simulink library "SelectiveChannelMuteBtc"  (R2022b)
settings: Solver=VariableStepAuto  StartTime=0.0  StopTime=10.0  RelTol=1e-3
libraries: TuneVar x3, $bdroot x2, RTC x2, FeaturePath x1, HandyTextFile x1, RgainyBtc x1
settings Model: Creator=kl13806  LastModifiedBy=kl13806
settings SolverCC: AlgebraicLoopSolver=TrustRegion
settings DebuggingCC: UnconnectedInputMsg=warning  UnconnectedOutputMsg=warning  UnconnectedLineMsg=warning  SFMachineParentedDataDiag=warning
settings ModelReferenceCC: EnableRefExpFcnMdlSchedulingChecks=on
settings RTWCC: DLArmComputeVersion=19.05

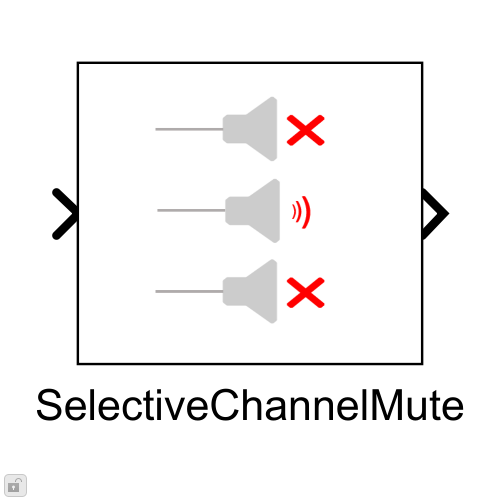
[thumbnail: Simulink's stored preview of the top-level diagram]
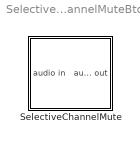
== system SelectiveChannelMuteBtc ==
  SelectiveChannelMute : Subsystem  mask(Bose Selective Channel Mute){Config=[], FeatureName=SCMute}
      mask prompts: Config "SelectiveChannelMuteConfig"; FeatureName "Feature path name:"
      mask help: This block offers the ability to mute individual channels selctively, by way of RGAINY and a "mute map". Set the initial mute state to a logical 1 (all channels muted) or 0 (no channels muted). There is runtime support via an RTC to selectively mute channels.
      mask init:
      | blkh=gcbh;
      | Config=BTConfig.Assert(blkh,Config);
      | Config.Validate();
      | BTConfig.InitSetFeatureIfPresent(blkh,'FeatureName');
      | 
      | 
      | MaskNumChannels = Config.NumChannelsIn;
      | 
      | % Set boundary conditions
      | rampRateBounds = [5,50000];
      | rampTimeBounds = [1,3000];
      mask Help:
      | This block offers the ability to mute individual channels seelctively, by way or RGAINY and a "mute map". Set the initial mute state to a logical 1 (all channels muted) or 0 (no channels muted). There is runtime support via an RTC to selectively mute channels.
      | 
      | RTC CONTROL:
      | Run time control is available to dynamically mute the audio of individual channels. The mute status can be provided to each channel through an array named "mute map". This array will be size 1 by numberOfInputChannels, and the elements of the array will be 1's (mute) or 0's (unmute), along with a ramp time and rate (rate gets precedence).
      | RTC_SIM_OBJ.AddREQ( 'SelectiveChannelMuteSet', 0.6, [0005,  <muteMap>, <ramp_db_per_second>, <ramp_time>]);
      | E.g., RTC_SIM_OBJ.AddREQ( 'MuteSet', 0.7, [0002, [1 0 0 1 0], 0, 50]);   % This message will mute channels 1 and 4 while keeping 2, 3, and 5 unmuted, all with a ramp time of 50 msec.
      mask Callback Config: BTConfig.CallbackHideIfPresent(gcbh,{'FeatureName'});
      mask TypeOptions FeatureName: FeaturePath/FeatureName
      mask Display: image('SCMuteIcon.png');

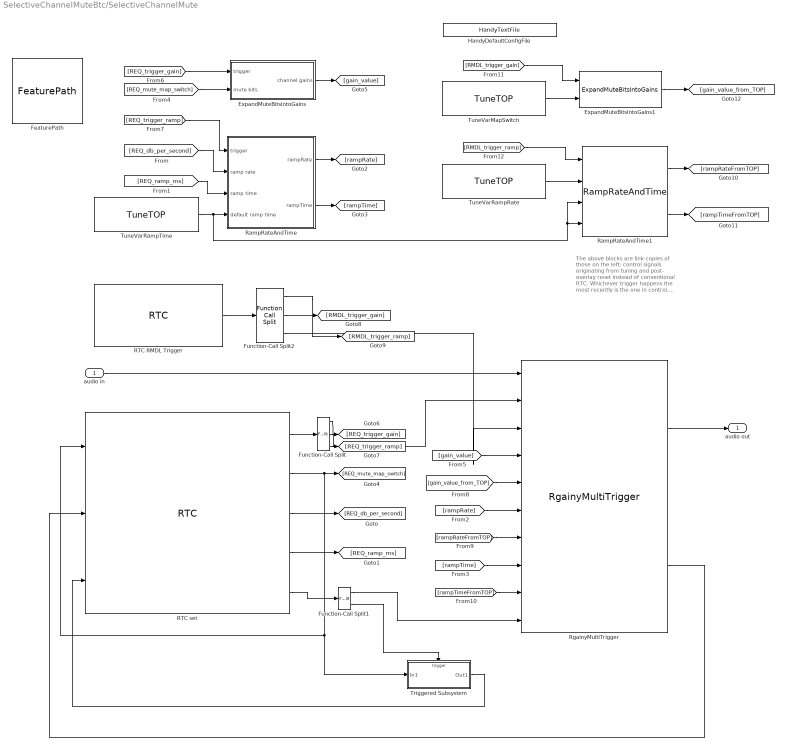
== system SelectiveChannelMuteBtc/SelectiveChannelMute ==
  note: The above blocks are link-copies
      | of those on the left: control signals
      | originating from tuning and post-
      | overlay reset instead of conventional
      | RTC. Whichever trigger happens the
      | most recently is the one in control.
      | (Note this design likely violates
      | standard RTC control assumptions)
  audio in : Inport
  ExpandMuteBitsIntoGains : Subsystem
  ExpandMuteBitsIntoGains1 : $bdroot/SelectiveChannelMute/ExpandMuteBitsIntoGains  SystemSampleTime=-1  VariantActivationTime=update diagram  Latency=0  AutoFrameSizeCalculation=off
  FeaturePath : FeaturePath/FeaturePath  FeatureName=SCMute  IsGroup=off  GroupNumber=-1  IsModule=off  TriggerInit=[20 -346 135 -239]
      settings: SourceProductName=Bose Talaria
  Function-Call Split : FunctionCallSplit  IconShape=distinctive  NumOutputPorts=3
  Function-Call Split1 : FunctionCallSplit  IconShape=distinctive  NumOutputPorts=2  OutputPortLayout=default
  Function-Call Split2 : FunctionCallSplit  IconShape=distinctive  NumOutputPorts=3
  HandyDefaultConfigFile : HandyTextFile/HandyTextFile  TemplateSource=Config  FileSuffix=Init  OpenDialogOnLoad=off  UseThisBlockName=off  AddGrandParentNamePrefix=off  TheDefaultText=|  ShowInLibBrowser=on
      | % $(FILENAME) Setup model parameters for each "Init" callback (e.g. update diagram)
      | sample_rate_in_hertz = 44100;
      | frame_size = 32;
      | sysin_channel_count = 2;
      settings: SourceProductName=Bose Talaria
  RTC RMDL Trigger : RTC/RTC  REQ_Priority=RTC_Mask.NormalPriority  RequestAtInit=off  EnableRequest=on  REQElemType1=uint32  REQElemWidth1=1  REQElemInitial1=[]  REQElemType2=uint32  REQElemWidth2=1  REQElemInitial2=[]  REQElemType3=uint32  REQElemWidth3=1  REQElemInitial3=[]  REQElemType4=uint32  REQElemWidth4=1  REQElemInitial4=[]  REQElemType5=uint32  REQElemWidth5=1  REQElemInitial5=[]  REQElemType6=uint32  REQElemWidth6=1  REQElemInitial6=[]  REQElemType7=uint32  REQElemWidth7=1  REQElemInitial7=[]  REQElemType8=uint32  REQElemWidth8=1  REQElemInitial8=[]  REQElemType9=uint32  REQElemWidth9=1  REQElemInitial9=[]  REQElemType10=uint32  REQElemWidth10=1  REQElemInitial10=[]  EnableResponse=on  EnableRSP_StatusIn=off  RSPElemType1=uint32  RSPElemWidth1=1  RSPElemType2=uint32  RSPElemWidth2=1  RSPElemType3=uint32  RSPElemWidth3=1  RSPElemType4=uint32  RSPElemWidth4=1  RSPElemType5=uint32  RSPElemWidth5=1  RSPElemType6=uint32  RSPElemWidth6=1  RSPElemType7=uint32  RSPElemWidth7=1  RSPElemType8=uint32  RSPElemWidth8=1  RSPElemType9=uint32  RSPElemWidth9=1  RSPElemType10=uint32  RSPElemWidth10=1  EnableNotification=off  EnableNTF_PrepTrig=off  NTFElemType1=uint32  NTFElemWidth1=1  NTFElemType2=uint32  NTFElemWidth2=1  NTFElemType3=uint32  NTFElemWidth3=1  NTFElemType4=uint32  NTFElemWidth4=1  NTFElemType5=uint32  NTFElemWidth5=1  NTFElemType6=uint32  NTFElemWidth6=1  NTFElemType7=uint32  NTFElemWidth7=1  NTFElemType8=uint32  NTFElemWidth8=1  NTFElemType9=uint32  NTFElemWidth9=1  NTFElemType10=uint32  NTFElemWidth10=1  MaskMessageName=RMDLTrigger
      settings: SourceProductName=Bose Talaria
  RTC set : RTC/RTC  Description="Command a mute by specifying whether mute is active (non zero mute_switch) or inactive (mute_switch is \"0\"). If db_per_second is non-zero, it commands the timing of the mute, otherwise the ramp_milliseconds is used."  REQ_Priority=RTC_Mask.NormalPriority  RequestAtInit=off  EnableRequest=on  REQElemName1=mute_map  REQElemType1=uint32  REQElemWidth1=1  REQElemInitial1=[]  REQElemName2=ramp_db_per_second  REQElemType2=uint32  REQElemWidth2=1  REQElemInitial2=[]  REQElemName3=ramp_milliseconds  REQElemType3=uint32  REQElemWidth3=1  REQElemInitial3=[]  REQElemType4=uint32  REQElemWidth4=1  REQElemInitial4=[]  REQElemType5=uint32  REQElemWidth5=1  REQElemInitial5=[]  REQElemType6=uint32  REQElemWidth6=1  REQElemInitial6=[]  REQElemType7=uint32  REQElemWidth7=1  REQElemInitial7=[]  REQElemType8=uint32  REQElemWidth8=1  REQElemInitial8=[]  REQElemType9=uint32  REQElemWidth9=1  REQElemInitial9=[]  REQElemType10=uint32  REQElemWidth10=1  REQElemInitial10=[]  EnableResponse=on  EnableRSP_StatusIn=off  RSPElemName1=mute_map  RSPElemType1=uint32  RSPElemWidth1=1  RSPElemType2=uint32  RSPElemWidth2=1  RSPElemType3=uint32  RSPElemWidth3=1  RSPElemType4=uint32  RSPElemWidth4=1  RSPElemType5=uint32  RSPElemWidth5=1  RSPElemType6=uint32  RSPElemWidth6=1  RSPElemType7=uint32  RSPElemWidth7=1  RSPElemType8=uint32  RSPElemWidth8=1  RSPElemType9=uint32  RSPElemWidth9=1  RSPElemType10=uint32  RSPElemWidth10=1  EnableNotification=on  EnableNTF_PrepTrig=off  NTFElemName1=mute_map  NTFElemType1=uint32  NTFElemWidth1=1  NTFElemType2=uint32  NTFElemWidth2=1  NTFElemType3=uint32  NTFElemWidth3=1  NTFElemType4=uint32  NTFElemWidth4=1  NTFElemType5=uint32  NTFElemWidth5=1  NTFElemType6=uint32  NTFElemWidth6=1  NTFElemType7=uint32  NTFElemWidth7=1  NTFElemType8=uint32  NTFElemWidth8=1  NTFElemType9=uint32  NTFElemWidth9=1  NTFElemType10=uint32  NTFElemWidth10=1  MaskMessageName=Set
      settings: SourceProductName=Bose Talaria
  RampRateAndTime : Subsystem
  RampRateAndTime1 : $bdroot/SelectiveChannelMute/RampRateAndTime  SystemSampleTime=-1  VariantActivationTime=update diagram  Latency=0  AutoFrameSizeCalculation=off
  RgainyMultiTrigger : RgainyBtc/RgainyMultiTrigger  GainOutEnable=off  Config=Config.Rgainy
      settings: SourceProductName=Bose Blocklib
  Triggered Subsystem : Subsystem  TreatAsAtomicUnit=on
  TuneVarMapSwitch : TuneVar/TuneTOP  TriggerInit=[725 -308 895 -252]  TopName=MapSwitch  TuneName=MapSwitch  DataType=single  TunabilityNumber=1  MinValue=[]  MaxValue=[]  BankNumber=0  PreOverlay=false  PostOverlay=false  UseSameName=on  MaskValue=Config.DefaultMuteBits
      settings: SourceProductName=Bose Talaria
  TuneVarRampRate : TuneVar/TuneTOP  TriggerInit=[725 -173 895 -117]  TopName=RampRate  TuneName=RampRate  DataType=single  TunabilityNumber=1  MinValue=[]  MaxValue=[]  BankNumber=0  PreOverlay=false  PostOverlay=false  UseSameName=on  MaskValue=Config.DefaultRampRateDbPerSec
      settings: SourceProductName=Bose Talaria
  TuneVarRampTime : TuneVar/TuneTOP  Description=|  TriggerInit=[155 -118 325 -62]  TopName=RampTime  TuneName=RampTime  DataType=single  TunabilityNumber=1  MinValue=1  MaxValue=100000  BankNumber=0  PreOverlay=false  PostOverlay=false  UseSameName=on  MaskValue=Config.DefaultRampTimeMsec
      | Specifies the default value of ramp time for the Mute or Unmute operation.
      | Used only when the RTC message does not contain either ramp rate or ramp time.
      settings: SourceProductName=Bose Talaria
  audio out : Outport  VectorParamsAs1DForOutWhenUnconnected=off
  wires:
  Triggered Subsystem/1(Out1) -> RTC set/3
  Function-Call Split1/2 -> Triggered Subsystem/Trigger
  Function-Call Split1/1 -> RgainyMultiTrigger/10
  RTC set/5 -> Function-Call Split1/1
  Function-Call Split/1 -> [REQ_trigger_ramp]
  Function-Call Split/2 -> [REQ_trigger_gain]
  [gain_value] -> RgainyMultiTrigger/4
  RTC set/2 -> [REQ_mute_map_switch], Triggered Subsystem/1(In1), RTC set/1
  [rampTime] -> RgainyMultiTrigger/8
  RTC set/4 -> [REQ_ramp_ms]
  [rampRate] -> RgainyMultiTrigger/6
  RTC set/3 -> [REQ_db_per_second]
  Function-Call Split/3 -> RgainyMultiTrigger/2
  RTC set/1 -> Function-Call Split/1
  audio in/1 -> RgainyMultiTrigger/1
  RgainyMultiTrigger/2 -> RTC set/2
  RgainyMultiTrigger/1 -> audio out/1
  Function-Call Split2/1 -> [RMDL_trigger_ramp]
  RTC RMDL Trigger/1 -> Function-Call Split2/1
  Function-Call Split2/3 -> RgainyMultiTrigger/3
  Function-Call Split2/2 -> [RMDL_trigger_gain]
  TuneVarMapSwitch/1 -> ExpandMuteBitsIntoGains1/2
  [RMDL_trigger_ramp] -> RampRateAndTime1/1
  TuneVarRampTime/1 -> RampRateAndTime/4(default ramp time), RampRateAndTime1/3, RampRateAndTime1/4
  TuneVarRampRate/1 -> RampRateAndTime1/2
  ExpandMuteBitsIntoGains1/1 -> [gain_value_from_TOP]
  RampRateAndTime1/2 -> [rampTimeFromTOP]
  RampRateAndTime1/1 -> [rampRateFromTOP]
  [RMDL_trigger_gain] -> ExpandMuteBitsIntoGains1/1
  [gain_value_from_TOP] -> RgainyMultiTrigger/5
  [rampRateFromTOP] -> RgainyMultiTrigger/7
  [rampTimeFromTOP] -> RgainyMultiTrigger/9
  [REQ_trigger_ramp] -> RampRateAndTime/1(trigger)
  [REQ_db_per_second] -> RampRateAndTime/2(ramp rate)
  [REQ_ramp_ms] -> RampRateAndTime/3(ramp time)
  RampRateAndTime/1(rampRate) -> [rampRate]
  RampRateAndTime/2(rampTime) -> [rampTime]
  [REQ_trigger_gain] -> ExpandMuteBitsIntoGains/1(trigger)
  [REQ_mute_map_switch] -> ExpandMuteBitsIntoGains/2(mute bits)
  ExpandMuteBitsIntoGains/1(channel gains) -> [gain_value]

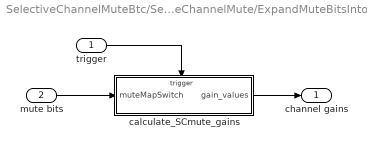
== system SelectiveChannelMuteBtc/SelectiveChannelMute/ExpandMuteBitsIntoGains ==
  trigger : Inport
  mute bits : Inport  Port=2
  calculate_SCmute_gains : MATLAB Function  TreatAsAtomicUnit=on
  channel gains : Outport
  wires:
  mute bits/1 -> calculate_SCmute_gains/1(muteMapSwitch)
  calculate_SCmute_gains/1(gain_values) -> channel gains/1
  trigger/1 -> calculate_SCmute_gains/Trigger

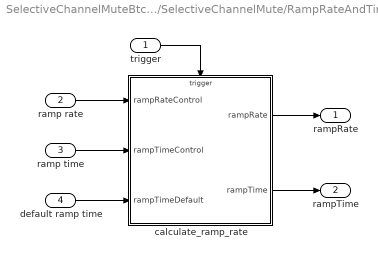
== system SelectiveChannelMuteBtc/SelectiveChannelMute/RampRateAndTime ==
  trigger : Inport
  ramp rate : Inport  Port=2
  ramp time : Inport  Port=3
  default ramp time : Inport  Port=4
  calculate_ramp_rate : MATLAB Function  TreatAsAtomicUnit=on
  rampRate : Outport
  rampTime : Outport  Port=2
  wires:
  trigger/1 -> calculate_ramp_rate/Trigger
  calculate_ramp_rate/2(rampTime) -> rampTime/1
  default ramp time/1 -> calculate_ramp_rate/3(rampTimeDefault)
  ramp rate/1 -> calculate_ramp_rate/1(rampRateControl)
  ramp time/1 -> calculate_ramp_rate/2(rampTimeControl)
  calculate_ramp_rate/1(rampRate) -> rampRate/1

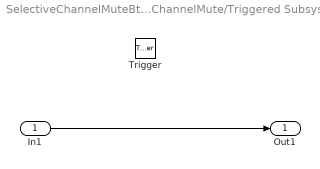
== system SelectiveChannelMuteBtc/SelectiveChannelMute/Triggered Subsystem ==
  In1 : Inport
  Trigger : TriggerPort  TriggerType=function-call  VariantControl=Variant
  Out1 : Outport
  wires:
  In1/1 -> Out1/1

== matlab function SelectiveChannelMuteBtc/SelectiveChannelMute/RampRateAndTime/calculate_ramp_rate ==
  data: rampRateControl input; rampRate output; rampTimeControl input; rampTime output; rampTimeDefault input; rampRateBounds parameter; rampTimeBounds parameter
  events: trigger input FUNCTION_CALL_EVENT
function [rampRate,rampTime] = Calculate_ramp_parameters(rampRateControl, rampTimeControl, rampTimeDefault,... % Inputs
    rampRateBounds, rampTimeBounds) % parameters

% Ramp time and rate are provided to the block as control signals. However 
% in case neither of them are provided (e.g. zero), the block will use the
% default ramp time provided separately often from a tune variable).

    rampTime = single(rampTimeDefault);
    rampRate = single(0);
    
    if (rampRateControl)
        rampRate = single(rampRateControl);
        rampRate = max(rampRateBounds(1), rampRate);
        rampRate = min(rampRateBounds(2), rampRate);
    end
    if (rampTimeControl)
        rampTime = single(rampTimeControl);
    end
    rampTime = max(rampTimeBounds(1), rampTime);
    rampTime = min(rampTimeBounds(2), rampTime);
end

== matlab function SelectiveChannelMuteBtc/SelectiveChannelMute/ExpandMuteBitsIntoGains/calculate_SCmute_gains ==
  data: muteMapSwitch input; gain_values output; MaskNumChannels parameter
  events: trigger input FUNCTION_CALL_EVENT
function gain_values = Calculate_SCMute_Gains(muteMapSwitch,MaskNumChannels)
%#codegen
% This function takes a uint32 and appropriates gain values to each
% channel, based on which channel has a 1 (muted) or 0 (unmuted).
% It works by doing a "bitand" operation, checking each bit against the
% binary representation of the muteMapSwitch that has been fed in from the
% RTC / Bam Proxy. Each bit represents a channel.
% Bit 1 = Channel 1, Bit 2 = Channel 2, Bit 3 = Channel, etc. 

gain_values = single(1.0) * ones(1,MaskNumChannels);

chanMask = uint32(1); % Set the bit to check against, starting at bit 1
muteMapSwitch = uint32(muteMapSwitch);
for chanNum = 1 : MaskNumChannels
    if bitand(muteMapSwitch,chanMask)
        gain_values(chanNum) = single(0.0);
    end
    % Move bit mask to the next bit (or "channel")
    chanMask = chanMask * 2;
end
